simulink model "FOCnew"  (R2024b)
settings: Solver=VariableStepAuto  StartTime=0.0  StopTime=2  RelTol=1e-3
libraries: slpidlib x3, simulink x3, spsDCVoltageSourceLib x2, spsThreePhaseVIMeasurementLib x1, spsThreeLevelBridgeLib x1, spsPermanentMagnetSynchronousMachineLib x1, spspowerguiLib x1
settings Model: Creator=GAUTHAM  LastModifiedBy=GAUTHAM
settings SolverCC: ZeroCrossAlgorithm=Adaptive
settings DebuggingCC: MaskedZcDiagnostic=none  IgnoredZcDiagnostic=none

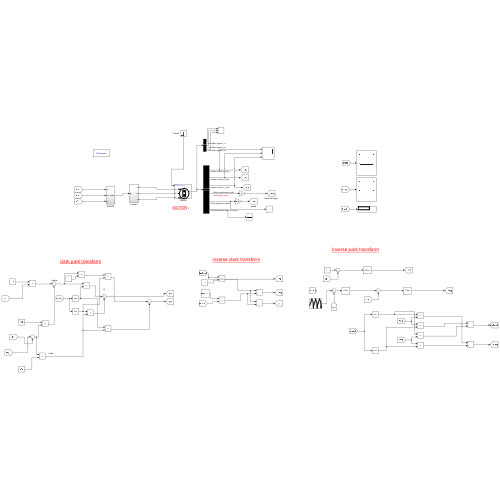
[thumbnail: Simulink's stored preview of the top-level diagram]
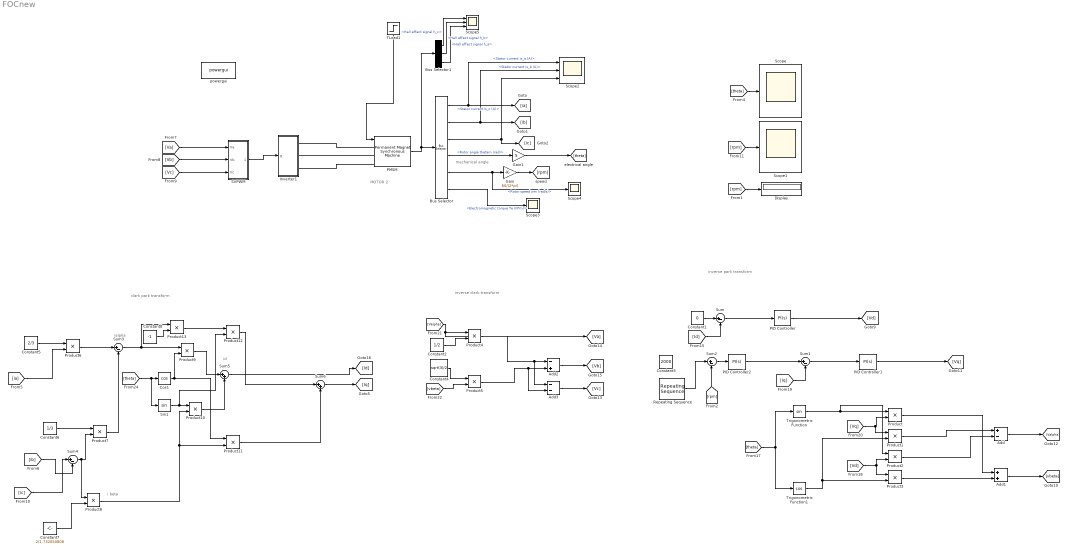
== system FOCnew ==
  note: MOTOR 2
  note: inverse park transform
  note: inverse clark transform
  note: clark park transform
  note: mechanical angle
  note: ialpha
  note: id
  note: i beta
  Add : Sum  Inputs=+-
  Add1 : Sum
  Add2 : Sum  Inputs=-+
  Add3 : Sum  Inputs=--
  Bus Selector : BusSelector  OutputSignals=Stator current is_a (A),Stator current is_b (A),Stator current is_c (A),Rotor angle thetam (rad),Rotor speed wm (rad/s),Electromagnetic torque Te (N*m)
  Bus Selector1 : BusSelector  OutputSignals=Hall effect signal h_c,Hall effect signal h_b,Hall effect signal h_a
  Constant1 : Constant  Value=0
  Constant2 : Constant  Value=1/2
  Constant3 : Constant  Value=2000
  Constant4 : Constant  Value=sqrt(3)/2
  Constant5 : Constant  Value=2/3
  Constant6 : Constant  Value=1/3
  Constant7 : Constant  Value=2/1.732050808
  Constant8 : Constant  Value=-1
  Cos1 : Trigonometry  Operator=cos
  Display : Display
  Gain : Gain  Gain=60/(2*pi)
  Gain1 : Gain  Gain=5
  Inverter1 : Subsystem
  PID Controller : slpidlib/PID Controller  Controller=PI  Form=Parallel  TimeDomain=Continuous-time  UseExternalTs=off  SampleTime=-1  IntegratorMethod=Forward Euler  FilterMethod=Forward Euler  ControllerParametersSource=internal  P=10  I=1  UseKiTs=off  D=0  UseExternalDerivativeSource=off  N=100  UseFilter=on  TunerSelectOption=Transfer Function Based (PID Tuner App)  InitialConditionSource=internal  InitialConditionForIntegrator=0  InitialConditionForFilter=0  DifferentiatorICPrevScaledInput=0  ExternalReset=none  TrackingMode=off  Kt=1  LimitOutput=off  SatLimitsSource=internal  UpperSaturationLimit=inf  LowerSaturationLimit=-inf  LinearizeAsGain=on  AntiWindupMode=none  Kb=1  LimitIntegrator=off  UpperIntegratorSaturationLimit=inf  LowerIntegratorSaturationLimit=-inf  POutMin=[]  POutMax=[]  IOutMin=[]  IOutMax=[]  DOutMin=[]  DOutMax=[]  NOutMin=[]  NOutMax=[]  SumOutMin=[]  SumOutMax=[]  SaturationOutMin=[]  SaturationOutMax=[]  PParamMin=[]  PParamMax=[]  IParamMin=[]  IParamMax=[]  DParamMin=[]  DParamMax=[]  NParamMin=[]  NParamMax=[]  KbParamMin=[]  KbParamMax=[]  KtParamMin=[]  KtParamMax=[]  KbOutMin=[]  KbOutMax=[]  KtOutMin=[]  KtOutMax=[]  IntegratorOutMin=[]  IntegratorOutMax=[]  FilterOutMin=[]  FilterOutMax=[]  SumI1OutMin=[]  SumI1OutMax=[]  SumI2OutMin=[]  SumI2OutMax=[]  SumI3OutMin=[]  SumI3OutMax=[]  SumI4OutMin=[]  SumI4OutMax=[]  SumDOutMin=[]  SumDOutMax=[]  DifferentiatorOutMin=[]  DifferentiatorOutMax=[]  FilterDiffOutCoefMin=[]  FilterDiffOutCoefMax=[]  ReciprocalOutMin=[]  ReciprocalOutMax=[]  SumDenOutMin=[]  SumDenOutMax=[]  SumNumOutMin=[]  SumNumOutMax=[]  DivideOutMin=[]  DivideOutMax=[]  UdiffTsProdOutMin=[]  UdiffTsProdOutMax=[]  NTsProdOutMin=[]  NTsProdOutMax=[]  UintegralTsProdOutMin=[]  UintegralTsProdOutMax=[]  UngainTsProdOutMin=[]  UngainTsProdOutMax=[]  ClampingZeroOutDataTypeStr=Inherit: Inherit via back propagation  ClampingZeroOutMin=[]  ClampingZeroOutMax=[]  FilterDenConstantOutDataTypeStr=Inherit: Inherit via back propagation  FilterDenConstantOutMin=[]  FilterDenConstantOutMax=[]  PCopyOutDataTypeStr=Inherit: Inherit via back propagation  PCopyOutMin=[]  PCopyOutMax=[]  NCopyOutDataTypeStr=Inherit: Inherit via back propagation  NCopyOutMin=[]  NCopyOutMax=[]  IntegratorContinuousStateAttributes=''  IntegratorStateMustResolveToSignalObject=off  IntegratorRTWStateStorageClass=Auto  FilterContinuousStateAttributes=''  FilterStateMustResolveToSignalObject=off  FilterRTWStateStorageClass=Auto  ParallelPVariant=InternalParameters  IdealPVariant=Disabled  IVariant=InternalParameters  DVariant=Disabled  IntegratorVariant=Continuous  SatVariant=Disabled  AWVariant=Passthrough  PCopyVariant=Disabled  TRVariant=Disabled  FdbkBlocksVariant=Forward  IdealPFdbkVariant=Disabled  SatFdbkVariant=Disabled  DerivativeFilterVariant=Disabled  NVariant=Disabled  NCopyVariant=Disabled_SignalSpec  FilterICVariant=Disabled  IntegratorICVariant=InternalICs  ExternalResetVariant=Disabled  TRSumVariant=Passthrough  SumFdbkVariant=Disabled  SumVariant=Sum_PI  TsampFilterVariant=InternalTs  TsampNgainVariant=Passthrough  TsampIntegralVariant=Disabled_SignalSpec  ExternalSaturationOutDataTypeStr=Inherit: Same as second input  DerivativeSourceVariant=Disabled  PreIntVariant=InternalPreInt
  PID Controller1 : slpidlib/PID Controller  Controller=PI  Form=Parallel  TimeDomain=Continuous-time  UseExternalTs=off  SampleTime=-1  IntegratorMethod=Forward Euler  FilterMethod=Forward Euler  ControllerParametersSource=internal  P=2  I=0.1  UseKiTs=off  D=0  UseExternalDerivativeSource=off  N=100  UseFilter=on  TunerSelectOption=Transfer Function Based (PID Tuner App)  InitialConditionSource=internal  InitialConditionForIntegrator=0  InitialConditionForFilter=0  DifferentiatorICPrevScaledInput=0  ExternalReset=none  TrackingMode=off  Kt=1  LimitOutput=off  SatLimitsSource=internal  UpperSaturationLimit=inf  LowerSaturationLimit=-inf  LinearizeAsGain=on  AntiWindupMode=none  Kb=1  LimitIntegrator=off  UpperIntegratorSaturationLimit=inf  LowerIntegratorSaturationLimit=-inf  POutMin=[]  POutMax=[]  IOutMin=[]  IOutMax=[]  DOutMin=[]  DOutMax=[]  NOutMin=[]  NOutMax=[]  SumOutMin=[]  SumOutMax=[]  SaturationOutMin=[]  SaturationOutMax=[]  PParamMin=[]  PParamMax=[]  IParamMin=[]  IParamMax=[]  DParamMin=[]  DParamMax=[]  NParamMin=[]  NParamMax=[]  KbParamMin=[]  KbParamMax=[]  KtParamMin=[]  KtParamMax=[]  KbOutMin=[]  KbOutMax=[]  KtOutMin=[]  KtOutMax=[]  IntegratorOutMin=[]  IntegratorOutMax=[]  FilterOutMin=[]  FilterOutMax=[]  SumI1OutMin=[]  SumI1OutMax=[]  SumI2OutMin=[]  SumI2OutMax=[]  SumI3OutMin=[]  SumI3OutMax=[]  SumI4OutMin=[]  SumI4OutMax=[]  SumDOutMin=[]  SumDOutMax=[]  DifferentiatorOutMin=[]  DifferentiatorOutMax=[]  FilterDiffOutCoefMin=[]  FilterDiffOutCoefMax=[]  ReciprocalOutMin=[]  ReciprocalOutMax=[]  SumDenOutMin=[]  SumDenOutMax=[]  SumNumOutMin=[]  SumNumOutMax=[]  DivideOutMin=[]  DivideOutMax=[]  UdiffTsProdOutMin=[]  UdiffTsProdOutMax=[]  NTsProdOutMin=[]  NTsProdOutMax=[]  UintegralTsProdOutMin=[]  UintegralTsProdOutMax=[]  UngainTsProdOutMin=[]  UngainTsProdOutMax=[]  ClampingZeroOutDataTypeStr=Inherit: Inherit via back propagation  ClampingZeroOutMin=[]  ClampingZeroOutMax=[]  FilterDenConstantOutDataTypeStr=Inherit: Inherit via back propagation  FilterDenConstantOutMin=[]  FilterDenConstantOutMax=[]  PCopyOutDataTypeStr=Inherit: Inherit via back propagation  PCopyOutMin=[]  PCopyOutMax=[]  NCopyOutDataTypeStr=Inherit: Inherit via back propagation  NCopyOutMin=[]  NCopyOutMax=[]  IntegratorContinuousStateAttributes=''  IntegratorStateMustResolveToSignalObject=off  IntegratorRTWStateStorageClass=Auto  FilterContinuousStateAttributes=''  FilterStateMustResolveToSignalObject=off  FilterRTWStateStorageClass=Auto  ParallelPVariant=InternalParameters  IdealPVariant=Disabled  IVariant=InternalParameters  DVariant=Disabled  IntegratorVariant=Continuous  SatVariant=Disabled  AWVariant=Passthrough  PCopyVariant=Disabled  TRVariant=Disabled  FdbkBlocksVariant=Forward  IdealPFdbkVariant=Disabled  SatFdbkVariant=Disabled  DerivativeFilterVariant=Disabled  NVariant=Disabled  NCopyVariant=Disabled_SignalSpec  FilterICVariant=Disabled  IntegratorICVariant=InternalICs  ExternalResetVariant=Disabled  TRSumVariant=Passthrough  SumFdbkVariant=Disabled  SumVariant=Sum_PI  TsampFilterVariant=InternalTs  TsampNgainVariant=Passthrough  TsampIntegralVariant=Disabled_SignalSpec  ExternalSaturationOutDataTypeStr=Inherit: Same as second input  DerivativeSourceVariant=Disabled  PreIntVariant=InternalPreInt
  PID Controller2 : slpidlib/PID Controller  Controller=PI  Form=Parallel  TimeDomain=Continuous-time  UseExternalTs=off  SampleTime=-1  IntegratorMethod=Forward Euler  FilterMethod=Forward Euler  ControllerParametersSource=internal  P=10  I=0.1  UseKiTs=off  D=0  UseExternalDerivativeSource=off  N=100  UseFilter=on  TunerSelectOption=Transfer Function Based (PID Tuner App)  InitialConditionSource=internal  InitialConditionForIntegrator=0  InitialConditionForFilter=0  DifferentiatorICPrevScaledInput=0  ExternalReset=none  TrackingMode=off  Kt=1  LimitOutput=off  SatLimitsSource=internal  UpperSaturationLimit=inf  LowerSaturationLimit=-inf  LinearizeAsGain=on  AntiWindupMode=none  Kb=1  LimitIntegrator=off  UpperIntegratorSaturationLimit=inf  LowerIntegratorSaturationLimit=-inf  POutMin=[]  POutMax=[]  IOutMin=[]  IOutMax=[]  DOutMin=[]  DOutMax=[]  NOutMin=[]  NOutMax=[]  SumOutMin=[]  SumOutMax=[]  SaturationOutMin=[]  SaturationOutMax=[]  PParamMin=[]  PParamMax=[]  IParamMin=[]  IParamMax=[]  DParamMin=[]  DParamMax=[]  NParamMin=[]  NParamMax=[]  KbParamMin=[]  KbParamMax=[]  KtParamMin=[]  KtParamMax=[]  KbOutMin=[]  KbOutMax=[]  KtOutMin=[]  KtOutMax=[]  IntegratorOutMin=[]  IntegratorOutMax=[]  FilterOutMin=[]  FilterOutMax=[]  SumI1OutMin=[]  SumI1OutMax=[]  SumI2OutMin=[]  SumI2OutMax=[]  SumI3OutMin=[]  SumI3OutMax=[]  SumI4OutMin=[]  SumI4OutMax=[]  SumDOutMin=[]  SumDOutMax=[]  DifferentiatorOutMin=[]  DifferentiatorOutMax=[]  FilterDiffOutCoefMin=[]  FilterDiffOutCoefMax=[]  ReciprocalOutMin=[]  ReciprocalOutMax=[]  SumDenOutMin=[]  SumDenOutMax=[]  SumNumOutMin=[]  SumNumOutMax=[]  DivideOutMin=[]  DivideOutMax=[]  UdiffTsProdOutMin=[]  UdiffTsProdOutMax=[]  NTsProdOutMin=[]  NTsProdOutMax=[]  UintegralTsProdOutMin=[]  UintegralTsProdOutMax=[]  UngainTsProdOutMin=[]  UngainTsProdOutMax=[]  ClampingZeroOutDataTypeStr=Inherit: Inherit via back propagation  ClampingZeroOutMin=[]  ClampingZeroOutMax=[]  FilterDenConstantOutDataTypeStr=Inherit: Inherit via back propagation  FilterDenConstantOutMin=[]  FilterDenConstantOutMax=[]  PCopyOutDataTypeStr=Inherit: Inherit via back propagation  PCopyOutMin=[]  PCopyOutMax=[]  NCopyOutDataTypeStr=Inherit: Inherit via back propagation  NCopyOutMin=[]  NCopyOutMax=[]  IntegratorContinuousStateAttributes=''  IntegratorStateMustResolveToSignalObject=off  IntegratorRTWStateStorageClass=Auto  FilterContinuousStateAttributes=''  FilterStateMustResolveToSignalObject=off  FilterRTWStateStorageClass=Auto  ParallelPVariant=InternalParameters  IdealPVariant=Disabled  IVariant=InternalParameters  DVariant=Disabled  IntegratorVariant=Continuous  SatVariant=Disabled  AWVariant=Passthrough  PCopyVariant=Disabled  TRVariant=Disabled  FdbkBlocksVariant=Forward  IdealPFdbkVariant=Disabled  SatFdbkVariant=Disabled  DerivativeFilterVariant=Disabled  NVariant=Disabled  NCopyVariant=Disabled_SignalSpec  FilterICVariant=Disabled  IntegratorICVariant=InternalICs  ExternalResetVariant=Disabled  TRSumVariant=Passthrough  SumFdbkVariant=Disabled  SumVariant=Sum_PI  TsampFilterVariant=InternalTs  TsampNgainVariant=Passthrough  TsampIntegralVariant=Disabled_SignalSpec  ExternalSaturationOutDataTypeStr=Inherit: Same as second input  DerivativeSourceVariant=Disabled  PreIntVariant=InternalPreInt
  PMSM : spsPermanentMagnetSynchronousMachineLib/Permanent Magnet Synchronous Machine  NbPhases=3  FluxDistribution=Sinusoidal  RotorType=Salient-pole  MechanicalLoad=Torque Tm  PresetModel=No  ShowDetailedParameters=on  MeasurementBus=off  Resistance=18.7  Inductance=8.5e-3  dqInductances=[0.02682 0.02682]  La=0.000395  MachineConstant=Flux linkage established by magnets (V.s)  Flux=0.18  VoltageCst=130.5936  TorqueCst=1.08  Flat=120  Mechanical=[0.0008 0 4 0]  PolePairs=2  InitialConditions=[0,0, 0,0]  InitialConditions5ph=[0 0 0 0 0 0]  RefAngle=90 degrees behind phase A axis (modified Park)  IterativeDiscreteModel=Trapezoidal non iterative  TsBlock=-1  TsPowergui=0
  Product{,1..13} (14 alike) : Product
  Repeating Sequence : simulink/Sources/Repeating Sequence  rep_seq_t=[0 0.2 0.3 0.4 0.5 0.6 0.8 0.9 1.0 1.2 1.4 1.6 1.8 2]  rep_seq_y=[500 500 800 800 1000 1000 1200 1500 1500 1800 1400 1400 1200 0]
  SVPWM : Subsystem
  Scope{,1,3..4} (4 alike) : Scope
  Scope2 : Scope  NumInputPorts=3
  Scope5 : Scope  NumInputPorts=3
  Sin1 : Trigonometry
  Sum{,1..4} (5 alike) : Sum  Inputs=|+-
  Sum5 : Sum  Inputs=|++
  Sum6 : Sum  Inputs=|++
  TLoad1 : Step  Time=0.1  Before=1  SampleTime=0
  Trigonometric Function : Trigonometry
  Trigonometric Function1 : Trigonometry  Operator=cos
  powergui : spspowerguiLib/powergui  Priority=1  SimulationMode=Continuous  SampleTime=50e-6  frequency=60  Iterations=50  frequencyindice=0  Pbase=100e6  ErrMax=1e-4  UnitsV=kV  UnitsW=MW  buscounter=0  FunctionMessages=off  echomessages=off  EnableUseOfTLC=off  CurrentSourceSwitches=off  DisableSnubberDevices=off  DisableRonSwitches=off  DisableVfSwitches=off  DisplayEquations=off  AutomaticDiscreteSolvers=off  SolverType=Tustin/Backward Euler (TBE)  Interpol=off  ExternalGateDelay=off  methode=off  Ts=100  x0status=blocks  SPID=on  SwTol=0  HookPort=off  NonlinearTolerance=1e-4  nMaxIteration=100  ContinueOnMaxIteration=off  RestoreLinks=warning  ResistiveCurrentMeasurement=off  Frange=[0:2:500]  Ylog=off  Xlog=on  ShowGrid=off  save=off  variable=ZData  structure=0  ZoomFFT=off  StartTime=0.0  cycles=1  DisplayStyle=1  fundamental=60  FreqAxis=off  MaxFrequency=1000  frequencyindicesteady=1  RmsSteady=1  display=off
  wires:
  Bus Selector/1 -> [ia], Scope2/1  "<Stator current is_a (A)>"
  Bus Selector/2 -> [ib], Scope2/2  "<Stator current is_b (A)>"
  Bus Selector/3 -> [ic], Scope2/3  "<Stator current is_c (A)>"
  Bus Selector/5 -> Scope4/1, Gain/1  "<Rotor speed wm (rad/s)>"
  Gain/1 -> [rpm]
  Bus Selector/4 -> Gain1/1  "<Rotor angle thetam (rad)>"
  Gain1/1 -> [theta]
  [theta] -> Scope/1
  [rpm] -> Scope1/1
  Constant2/1 -> Product4/2
  [vbeta] -> Product5/2
  Product5/1 -> Add3/2, Add2/2
  Add3/1 -> [Vc]
  Constant4/1 -> Product5/1
  Product4/1 -> Add3/1, Add2/1
  [Valpha] -> [Va], Product4/1
  Add2/1 -> [Vb]
  Product3/1 -> Add1/2
  Product/1 -> Add1/1
  PID Controller/1 -> [Vd]
  [Id] -> Sum/2
  Trigonometric Function1/1 -> Product3/2, Product1/2
  PID Controller1/1 -> [Vq]
  Trigonometric Function/1 -> Product2/1, Product/1
  [rpm] -> Sum2/2
  [Vq] -> Product1/1, Product/2
  PID Controller2/1 -> Sum1/1
  Constant1/1 -> Sum/1
  [Vd] -> Product3/1, Product2/2
  Sum2/1 -> PID Controller2/1
  [theta] -> Trigonometric Function1/1, Trigonometric Function/1
  Product1/1 -> Add/1
  Product2/1 -> Add/2
  Add/1 -> [Valpha]
  Sum/1 -> PID Controller/1
  Add1/1 -> [vbeta]
  [Iq] -> Sum1/2
  Sum1/1 -> PID Controller1/1
  Constant8/1 -> Product13/2
  Product6/1 -> Sum3/1
  [theta] -> Sin1/1, Cos1/1
  Product11/1 -> Sum6/2
  Product12/1 -> Sum6/1
  Sum4/1 -> Product8/1, Product7/2
  Product7/1 -> Sum3/2
  Sin1/1 -> Product12/2, Product10/1
  Sum6/1 -> [Iq]
  [ic] -> Sum4/1
  Constant6/1 -> Product7/1
  Product8/1 -> Product11/2, Product10/2
  Sum3/1 -> Product13/1, Product9/1
  [ib] -> Sum4/2
  Constant5/1 -> Product6/1
  Product10/1 -> Sum5/2
  Constant7/1 -> Product8/2
  Cos1/1 -> Product9/2, Product11/1
  Product13/1 -> Product12/1
  [ia] -> Product6/2
  Product9/1 -> Sum5/1
  Sum5/1 -> [Id]
  Bus Selector/6 -> Scope3/1  "<Electromagnetic torque Te (N*m)>"
  [Va] -> SVPWM/1(Va)
  [Vb] -> SVPWM/2(Vb)
  [Vc] -> SVPWM/3(Vc)
  SVPWM/1(pulse) -> Inverter1/1(g)
  [rpm] -> Display/1
  Bus Selector1/1 -> Scope5/1  "<Hall effect signal h_c>"
  Bus Selector1/2 -> Scope5/2  "<Hall effect signal h_b>"
  Bus Selector1/3 -> Scope5/3  "<Hall effect signal h_a>"
  Repeating Sequence/1 -> Sum2/1
  TLoad1/1 -> PMSM/1
  PMSM/1 -> Bus Selector1/1, Bus Selector/1
  connections:
  PMSM/LConn1 -- Inverter1/RConn1
  PMSM/LConn2 -- Inverter1/RConn2
  PMSM/LConn3 -- Inverter1/RConn3

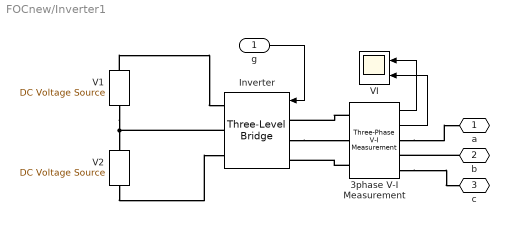
== system FOCnew/Inverter1 ==
  g : Inport
  3phase V-I Measurement : spsThreePhaseVIMeasurementLib/Three-Phase V-I Measurement  VoltageMeasurement=phase-to-phase  SetLabelV=off  LabelV=Vabc  Vpu=off  VpuLL=off  CurrentMeasurement=yes  SetLabelI=off  LabelI=Iabc  Ipu=off  Pbase=100e6  Vbase=500e3  OutputType=Complex  PhasorSimulation=off  PSBequivalent=0
  Inverter : spsThreeLevelBridgeLib/Three-Level Bridge  Arms=3  SnubberResistance=50  SbubberCapacitance=1e-6  Device=IGBT / Diodes  Ron=0.2e-3  ForwardVoltages="[  2 1 ]"  Measurements=All voltages and currents
      settings: AttributesFormatString=\n
  V1 : spsDCVoltageSourceLib/DC Voltage Source  Amplitude=36  Measurements=None
  V2 : spsDCVoltageSourceLib/DC Voltage Source  Amplitude=36  Measurements=None
  VI : Scope  NumInputPorts=2
  a : PMIOPort  Side=Right
  b : PMIOPort  Port=2  Side=Right
  c : PMIOPort  Port=3  Side=Right
  wires:
  3phase V-I Measurement/2 -> VI/2
  g/1 -> Inverter/1
  3phase V-I Measurement/1 -> VI/1
  connections:
  3phase V-I Measurement/LConn1 -- Inverter/LConn1
  V2/LConn1 -- Inverter/RConn3
  3phase V-I Measurement/LConn3 -- Inverter/LConn3
  Inverter/RConn2 -- V1/LConn1 -- V2/RConn1
  V1/RConn1 -- Inverter/RConn1
  Inverter/LConn2 -- 3phase V-I Measurement/LConn2
  3phase V-I Measurement/RConn3 -- c/RConn1
  b/RConn1 -- 3phase V-I Measurement/RConn2
  3phase V-I Measurement/RConn1 -- a/RConn1

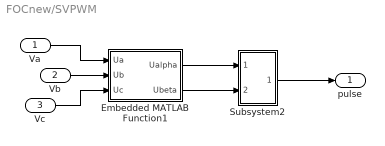
== system FOCnew/SVPWM ==
  Va : Inport
  Vb : Inport  Port=2
  Vc : Inport  Port=3
  Embedded MATLAB Function1 : MATLAB Function  TreatAsAtomicUnit=on
  Subsystem2 : Subsystem
  pulse : Outport
  wires:
  Embedded MATLAB Function1/2(Ubeta) -> Subsystem2/2(Ubeta)
  Subsystem2/1(pulse) -> pulse/1
  Vb/1 -> Embedded MATLAB Function1/2(Ub)
  Vc/1 -> Embedded MATLAB Function1/3(Uc)
  Embedded MATLAB Function1/1(Ualpha) -> Subsystem2/1(Ualfa)
  Va/1 -> Embedded MATLAB Function1/1(Ua)

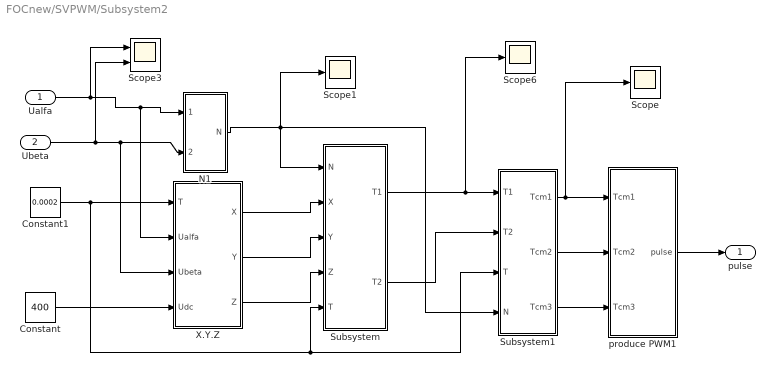
== system FOCnew/SVPWM/Subsystem2 ==
  Ualfa : Inport
  Ubeta : Inport  Port=2
  Constant : Constant  Value=400
  Constant1 : Constant  Value=0.0002
  N1 : Subsystem
  Scope : Scope
  Scope1 : Scope
  Scope3 : Scope  NumInputPorts=2
  Scope6 : Scope
  Subsystem : Subsystem
  Subsystem1 : Subsystem
  X.Y.Z : Subsystem
  produce PWM1 : Subsystem
  pulse : Outport
  wires:
  Constant1/1 -> X.Y.Z/1(T), Subsystem1/3(T), Subsystem/5(T)
  Constant/1 -> X.Y.Z/4(Udc)
  N1/1(N) -> Subsystem1/4(N), Scope1/1, Subsystem/1(N)
  X.Y.Z/1(X) -> Subsystem/2(X)
  X.Y.Z/2(Y) -> Subsystem/3(Y)
  X.Y.Z/3(Z) -> Subsystem/4(Z)
  Subsystem1/1(Tcm1) -> Scope/1, produce PWM1/1(Tcm1)
  Subsystem1/2(Tcm2) -> produce PWM1/2(Tcm2)
  Subsystem1/3(Tcm3) -> produce PWM1/3(Tcm3)
  Ualfa/1 -> Scope3/1, X.Y.Z/2(Ualfa), N1/1(Ualfa)
  Subsystem/1(T1) -> Subsystem1/1(T1), Scope6/1
  Subsystem/2(T2) -> Subsystem1/2(T2)
  Ubeta/1 -> N1/2(Ubeta), X.Y.Z/3(Ubeta), Scope3/2
  produce PWM1/1(pulse) -> pulse/1

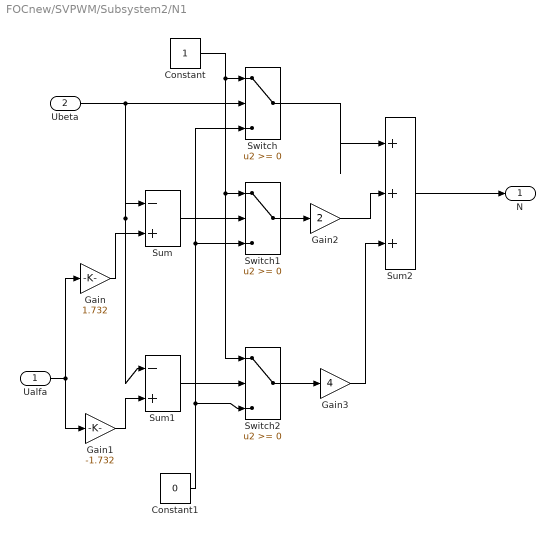
== system FOCnew/SVPWM/Subsystem2/N1 ==
  Ualfa : Inport
  Ubeta : Inport  Port=2
  Constant : Constant
  Constant1 : Constant  Value=0
  Gain : Gain  Gain=1.732
  Gain1 : Gain  Gain=-1.732
  Gain2 : Gain  Gain=2
  Gain3 : Gain  Gain=4
  Sum : Sum  Inputs=|-+
  Sum1 : Sum  Inputs=|-+
  Sum2 : Sum  Inputs=|+++
  Switch : Switch  SaturateOnIntegerOverflow=off  InputSameDT=off
  Switch1 : Switch  SaturateOnIntegerOverflow=off  InputSameDT=off
  Switch2 : Switch  SaturateOnIntegerOverflow=off  InputSameDT=off
  N : Outport
  wires:
  Ubeta/1 -> Switch/2, Sum/1, Sum1/1
  Constant/1 -> Switch/1, Switch2/1, Switch1/1
  Ualfa/1 -> Gain1/1, Gain/1
  Gain/1 -> Sum/2
  Sum/1 -> Switch1/2
  Sum1/1 -> Switch2/2
  Gain1/1 -> Sum1/2
  Constant1/1 -> Switch/3, Switch1/3, Switch2/3
  Switch1/1 -> Gain2/1
  Switch2/1 -> Gain3/1
  Gain2/1 -> Sum2/2
  Switch/1 -> Sum2/1
  Gain3/1 -> Sum2/3
  Sum2/1 -> N/1

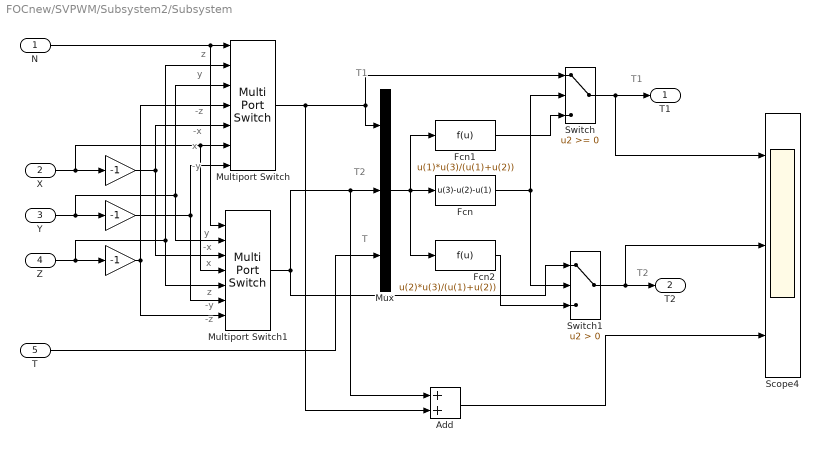
== system FOCnew/SVPWM/Subsystem2/Subsystem ==
  note: z
  note: y
  note: -z
  note: -x
  note: x
  note: -y
  note: y
  note: -x
  note: x
  note: z
  note: -y
  note: -z
  note: T1
  note: T2
  note: T
  note: T1
  note: T2
  N : Inport
  X : Inport  Port=2
  Y : Inport  Port=3
  Z : Inport  Port=4
  T : Inport  Port=5
  " " : Gain  Gain=-1
  "  " : Gain  Gain=-1
  "    " : Gain  Gain=-1
  Add : Sum
  Fcn : Fcn  Expr=u(3)-u(2)-u(1)
  Fcn1 : Fcn  Expr=u(1)*u(3)/(u(1)+u(2))
  Fcn2 : Fcn  Expr=u(2)*u(3)/(u(1)+u(2))
  Multiport Switch : MultiPortSwitch  Inputs=6  SaturateOnIntegerOverflow=off  InputSameDT=off
  Multiport Switch1 : MultiPortSwitch  Inputs=6  SaturateOnIntegerOverflow=off  InputSameDT=off
  Mux : Mux  Inputs=3
  Scope4 : Scope  NumInputPorts=3
  Switch : Switch  SaturateOnIntegerOverflow=off  InputSameDT=off
  Switch1 : Switch  Criteria=u2 > Threshold  SaturateOnIntegerOverflow=off  InputSameDT=off
  T1 : Outport
  T2 : Outport  Port=2
  wires:
  N/1 -> Multiport Switch1/1, Multiport Switch/1
  X/1 -> Multiport Switch1/4, Multiport Switch/6, " "/1
  Y/1 -> Multiport Switch1/2, Multiport Switch/3, "  "/1
  Z/1 -> Multiport Switch1/5, Multiport Switch/2, "    "/1
  "    "/1 -> Multiport Switch1/7, Multiport Switch/4
  "  "/1 -> Multiport Switch/7, Multiport Switch1/6
  " "/1 -> Multiport Switch/5, Multiport Switch1/3
  Multiport Switch/1 -> Mux/1, Switch/1, Add/2
  Multiport Switch1/1 -> Switch1/1, Mux/2, Add/1
  T/1 -> Mux/3
  Mux/1 -> Fcn/1, Fcn1/1, Fcn2/1
  Fcn/1 -> Switch/2, Switch1/2
  Fcn1/1 -> Switch/3
  Fcn2/1 -> Switch1/3
  Switch/1 -> T1/1, Scope4/1
  Switch1/1 -> T2/1, Scope4/2
  Add/1 -> Scope4/3

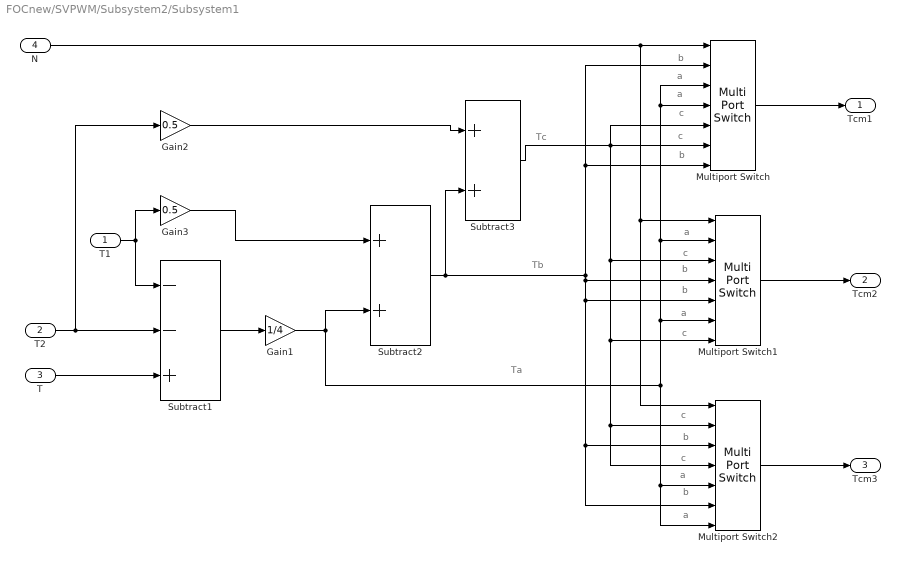
== system FOCnew/SVPWM/Subsystem2/Subsystem1 ==
  note: Ta
  note: Tb
  note: Tc
  note: b
  note: a
  note: a
  note: c
  note: c
  note: b
  note: a
  note: c
  note: b
  note: b
  note: a
  note: c
  note: c
  note: b
  note: c
  note: a
  note: b
  note: a
  T1 : Inport
  T2 : Inport  Port=2
  T : Inport  Port=3
  N : Inport  Port=4
  Gain1 : Gain  Gain=1/4
  Gain2 : Gain  Gain=0.5
  Gain3 : Gain  Gain=0.5
  Multiport Switch : MultiPortSwitch  Inputs=6  SaturateOnIntegerOverflow=off  InputSameDT=off
  Multiport Switch1 : MultiPortSwitch  Inputs=6  SaturateOnIntegerOverflow=off  InputSameDT=off
  Multiport Switch2 : MultiPortSwitch  Inputs=6  SaturateOnIntegerOverflow=off  InputSameDT=off
  Subtract1 : Sum  Inputs=--+
  Subtract2 : Sum
  Subtract3 : Sum
  Tcm1 : Outport
  Tcm2 : Outport  Port=2
  Tcm3 : Outport  Port=3
  wires:
  T2/1 -> Gain2/1, Subtract1/2
  T/1 -> Subtract1/3
  T1/1 -> Gain3/1, Subtract1/1
  Gain3/1 -> Subtract2/1
  Subtract1/1 -> Gain1/1
  Gain1/1 -> Subtract2/2, Multiport Switch/3, Multiport Switch/4, Multiport Switch1/2, Multiport Switch1/6, Multiport Switch2/5, Multiport Switch2/7
  Subtract2/1 -> Subtract3/2, Multiport Switch/2, Multiport Switch/7, Multiport Switch1/4, Multiport Switch1/5, Multiport Switch2/3, Multiport Switch2/6
  Gain2/1 -> Subtract3/1
  N/1 -> Multiport Switch/1, Multiport Switch2/1, Multiport Switch1/1
  Multiport Switch/1 -> Tcm1/1
  Multiport Switch1/1 -> Tcm2/1
  Multiport Switch2/1 -> Tcm3/1
  Subtract3/1 -> Multiport Switch/5, Multiport Switch/6, Multiport Switch1/3, Multiport Switch1/7, Multiport Switch2/2, Multiport Switch2/4

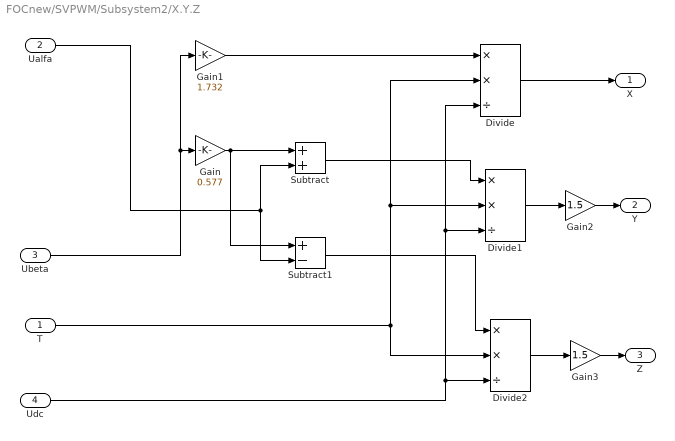
== system FOCnew/SVPWM/Subsystem2/X.Y.Z ==
  T : Inport
  Ualfa : Inport  Port=2
  Ubeta : Inport  Port=3
  Udc : Inport  Port=4
  Divide : Product  Inputs=**/
  Divide1 : Product  Inputs=**/
  Divide2 : Product  Inputs=**/
  Gain : Gain  Gain=0.577
  Gain1 : Gain  Gain=1.732
  Gain2 : Gain  Gain=1.5
  Gain3 : Gain  Gain=1.5
  Subtract : Sum
  Subtract1 : Sum  Inputs=+-
  X : Outport
  Y : Outport  Port=2
  Z : Outport  Port=3
  wires:
  Gain/1 -> Subtract/1, Subtract1/1
  Gain1/1 -> Divide/1
  T/1 -> Divide2/2, Divide1/2, Divide/2
  Udc/1 -> Divide2/3, Divide1/3, Divide/3
  Ualfa/1 -> Subtract1/2, Subtract/2
  Subtract/1 -> Divide1/1
  Subtract1/1 -> Divide2/1
  Divide/1 -> X/1
  Divide1/1 -> Gain2/1
  Divide2/1 -> Gain3/1
  Gain2/1 -> Y/1
  Gain3/1 -> Z/1
  Ubeta/1 -> Gain1/1, Gain/1

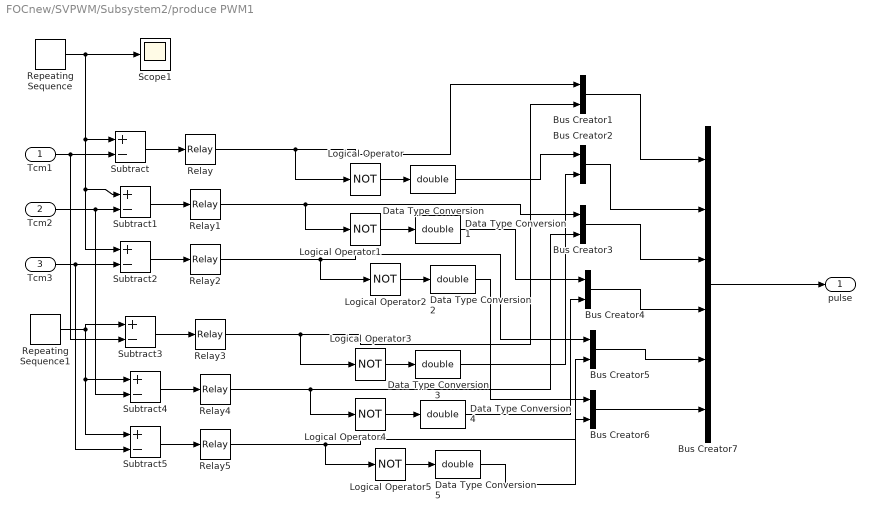
== system FOCnew/SVPWM/Subsystem2/produce PWM1 ==
  Tcm1 : Inport
  Tcm2 : Inport  Port=2
  Tcm3 : Inport  Port=3
  Bus Creator{1..6} (6 alike) : BusCreator  Inputs=2
  Bus Creator7 : BusCreator  Inputs=6
  Data Type Conversion{,1..5} (6 alike) : DataTypeConversion  OutDataTypeStr=double  SaturateOnIntegerOverflow=off  RndMeth=Floor
  Logical Operator{,1..5} (6 alike) : Logic  Operator=NOT  AllPortsSameDT=off
  Relay{,1..5} (6 alike) : Relay
  Repeating Sequence : simulink/Sources/Repeating Sequence  rep_seq_t=[0 0.0001 0.0002]  rep_seq_y=[0 0.0001/2 0]
  Repeating Sequence1 : simulink/Sources/Repeating Sequence  rep_seq_t=[0 0.0001 0.0002]  rep_seq_y=[0.0001/2 0.0001 0.0001/2]
  Scope1 : Scope
  Subtract{,1..5} (6 alike) : Sum  Inputs=+-
  pulse : Outport
  wires:
  Data Type Conversion2/1 -> Bus Creator6/1
  Data Type Conversion1/1 -> Bus Creator4/1
  Data Type Conversion/1 -> Bus Creator2/1
  Relay2/1 -> Logical Operator2/1, Bus Creator5/1
  Relay1/1 -> Logical Operator1/1, Bus Creator3/1
  Relay/1 -> Logical Operator/1, Bus Creator1/1
  Logical Operator/1 -> Data Type Conversion/1
  Logical Operator2/1 -> Data Type Conversion2/1
  Logical Operator1/1 -> Data Type Conversion1/1
  Tcm3/1 -> Subtract2/2, Subtract5/2
  Tcm2/1 -> Subtract1/2, Subtract4/2
  Tcm1/1 -> Subtract/2, Subtract3/2
  Repeating Sequence/1 -> Scope1/1, Subtract1/1, Subtract2/1, Subtract/1
  Subtract2/1 -> Relay2/1
  Subtract1/1 -> Relay1/1
  Subtract/1 -> Relay/1
  Subtract5/1 -> Relay5/1
  Subtract4/1 -> Relay4/1
  Subtract3/1 -> Relay3/1
  Repeating Sequence1/1 -> Subtract3/1, Subtract4/1, Subtract5/1
  Data Type Conversion5/1 -> Bus Creator6/2
  Data Type Conversion4/1 -> Bus Creator4/2
  Data Type Conversion3/1 -> Bus Creator2/2
  Relay5/1 -> Logical Operator5/1, Bus Creator5/2
  Relay4/1 -> Logical Operator4/1, Bus Creator3/2
  Relay3/1 -> Logical Operator3/1, Bus Creator1/2
  Logical Operator3/1 -> Data Type Conversion3/1
  Logical Operator5/1 -> Data Type Conversion5/1
  Logical Operator4/1 -> Data Type Conversion4/1
  Bus Creator1/1 -> Bus Creator7/1
  Bus Creator2/1 -> Bus Creator7/2
  Bus Creator3/1 -> Bus Creator7/3
  Bus Creator4/1 -> Bus Creator7/4
  Bus Creator5/1 -> Bus Creator7/5
  Bus Creator6/1 -> Bus Creator7/6
  Bus Creator7/1 -> pulse/1

== matlab function FOCnew/SVPWM/Embedded MATLAB Function1 ==
  settings: fimath=|
      | fimath(...
      | 'RoundMode', 'floor',...
      | 'OverflowMode', 'wrap',...
      | 'ProductMode', 'KeepLSB', 'ProductWordLength', 32,...
      | 'SumMode', 'KeepLSB', 'SumWordLength', 32,...
      | 'CastBeforeSum', false)
  data: Ua input; Ualpha output; Ub input; Uc input; Ubeta output
function [Ualpha,Ubeta]= fcn(Ua,Ub,Uc) 
Ualpha=2/3*(Ua-0.5*Ub-0.5*Uc);
Ubeta=2/3*(sqrt(3)/2*Ub-sqrt(3)/2*Uc);
